simulink model "multipath_fading"  (Simulink 5.0)
settings: Solver=ode45  StartTime=0.0  StopTime=1  RelTol=1e-3
undefined symbols (not defined in the file): get, p, y
libraries: dspmathops x40, dspstat3 x1, simulink x1, dspsnks4 x1
(part 2 of 2)

== system multipath_fading/path21 to path40, 20 paths/path31 to path40, 10 paths/path36 to path40, 5 paths/path40 ==
  note: initial phase
      | 0-2pi
      | uniformly
      | distributed
  note: incidence angle
      | 0-2pi
      | uniformity
      | distributed
  note: gain
      | 0-1uniformly distributed
  note: Fm_A
  Fm : Inport
  time : Inport  Port=2
  signal : Inport  Port=3
  Angle : Constant  Value=rand(1)*2*pi
  Complex Exponential4 : dspmathops/Complex Exponential
  Divide2 : Product  Inputs=**  OutScaling=2^-10
  Gain1 : Gain  Gain=rand(1)
  Phase : Constant  Value=rand(1)*2*pi
  Product1 : Product  RndMeth=Zero
  Product2 : Product  RndMeth=Zero
  Sum3 : Sum  Inputs=|--
  cos : Trigonometry  Operator=cos
  Out1 : Outport
  wires:
  Phase/1 -> Sum3/1
  Complex Exponential4/1 -> Gain1/1
  Sum3/1 -> Complex Exponential4/1  "Phase"
  Angle/1 -> cos/1
  Fm/1 -> Divide2/1
  cos/1 -> Divide2/2
  time/1 -> Product1/1
  Divide2/1 -> Product1/2
  Product1/1 -> Sum3/2
  Gain1/1 -> Product2/1
  Product2/1 -> Out1/1
  signal/1 -> Product2/2
